simulink model "bh_TH1_CONTROL_Dual_loop_POS_SETTLE_0p05_THETA_TRACK"  (R2016b)
settings: Solver=ode23t  StartTime=0.0  StopTime=60  RelTol=1e-5  EnableMultiTasking=on
values from neighbouring files (symbols this model uses):
  g = 9.80665    [bh_params_single_link_control_explore.m]
  L1x = 1.5    [bh_params_single_link_control_explore.m]
  L1y = 0.050    (= 0.05)    [bh_params_single_link_control_explore.m]
  L1z = 0.005    [bh_params_single_link_control_explore.m]
  mass1 = density * L1x*L1y*L1z    (= 0.375)    [bh_params_single_link_control_explore.m]
undefined symbols (not defined in the file or in its folder): X, Y, Z
libraries: sm_lib x6, nesl_utility x6, simulink_extras x3, simulink x2, discretizing x1
settings Model: Creator=bhorton  LastModifiedBy=bhorton
settings SolverCC: ZeroCrossAlgorithm=Adaptive
settings OptimizationCC: LifeSpan=inf
settings DebuggingCC: SFUnexpectedBacktrackingDiag=warning  SFNoUnconditionalDefaultTransitionDiag=warning  SFExecutionAtInitializationDiag=none
settings GRTTargetCC: TargetLangStandard=C89/C90 (ANSI)
settings ConfigComp: CovMetricSettings=dw  CovHtmlReporting=on  CovSaveCumulativeToWorkspaceVar=on  CovSaveSingleToWorkspaceVar=on  CovExternalEMLEnable=off
settings SimscapeCC: SimscapeLogType=all  SimscapeLogDataHistory=10000

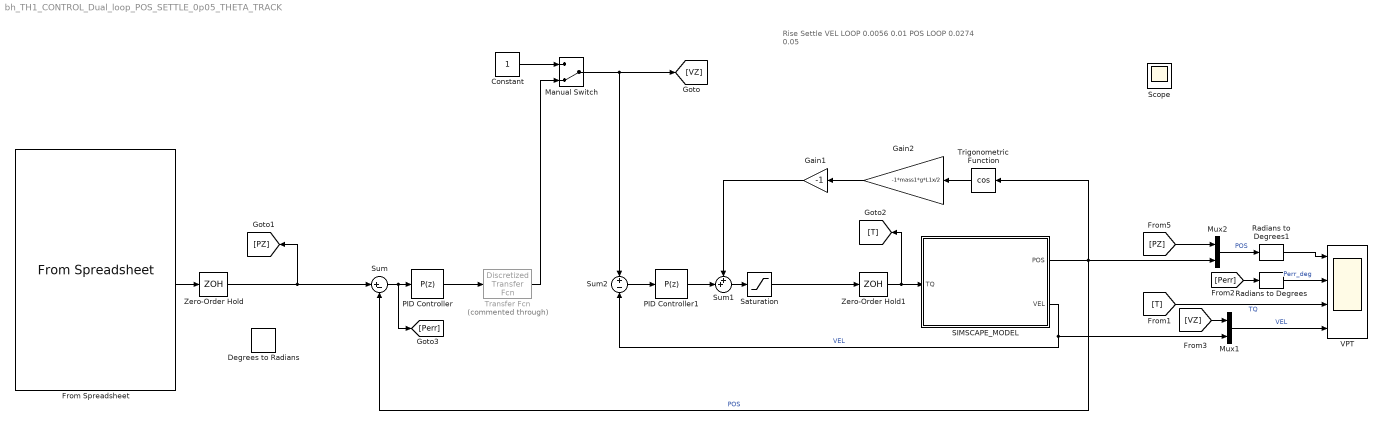
== system bh_TH1_CONTROL_Dual_loop_POS_SETTLE_0p05_THETA_TRACK ==
  note: Rise Settle
      | VEL LOOP 0.0056 0.01
      | POS LOOP 0.0274 0.05
  Constant : Constant
  Degrees to Radians : simulink_extras/Transformations/Degrees to Radians
  From Spreadsheet : FromSpreadsheet  FileName=bh_theta_data.xlsx  SheetName=THETA_SHEET  SampleTime=0.01  ExtrapolationBeforeFirstDataPoint=Hold first value  ExtrapolationAfterLastDataPoint=Hold last value
  Gain1 : Gain  Gain=-1
  Gain2 : Gain  Gain=-1*mass1*g*L1x/2
  Manual Switch : ManualSwitch  CurrentSetting=0
  Mux1 : Mux  Inputs=2
  Mux2 : Mux  Inputs=2
  PID Controller : simulink/Continuous/PID Controller  Controller=P  TimeDomain=Discrete-time  SampleTime=0.001  IntegratorMethod=Forward Euler  FilterMethod=Forward Euler  Form=Parallel  UseFilter=on  ControllerParametersSource=internal  P=63.9  I=3.94651136246193  D=0  N=100  InitialConditionSource=internal  InitialConditionForIntegrator=0  InitialConditionForFilter=0  ExternalReset=none  LimitOutput=off  UpperSaturationLimit=inf  LowerSaturationLimit=-inf  LinearizeAsGain=on  AntiWindupMode=none  Kb=1  TrackingMode=off  Kt=1  PParamMin=[]  PParamMax=[]  IParamMin=[]  IParamMax=[]  DParamMin=[]  DParamMax=[]  NParamMin=[]  NParamMax=[]  KbParamMin=[]  KbParamMax=[]  KtParamMin=[]  KtParamMax=[]  POutMin=[]  POutMax=[]  IOutMin=[]  IOutMax=[]  DOutMin=[]  DOutMax=[]  NOutMin=[]  NOutMax=[]  KbOutMin=[]  KbOutMax=[]  KtOutMin=[]  KtOutMax=[]  IntegratorOutMin=[]  IntegratorOutMax=[]  FilterOutMin=[]  FilterOutMax=[]  SumOutMin=[]  SumOutMax=[]  SumI1OutMin=[]  SumI1OutMax=[]  SumI2OutMin=[]  SumI2OutMax=[]  SumI3OutMin=[]  SumI3OutMax=[]  SumDOutMin=[]  SumDOutMax=[]  SaturationOutMin=[]  SaturationOutMax=[]  IntegratorContinuousStateAttributes=''  IntegratorStateMustResolveToSignalObject=off  IntegratorRTWStateStorageClass=Auto  FilterContinuousStateAttributes=''  FilterStateMustResolveToSignalObject=off  FilterRTWStateStorageClass=Auto  DifferentiatorICPrevScaledInput=0  DifferentiatorOutMin=[]  DifferentiatorOutMax=[]
  PID Controller1 : simulink/Continuous/PID Controller  Controller=P  TimeDomain=Discrete-time  SampleTime=0.001  IntegratorMethod=Forward Euler  FilterMethod=Forward Euler  Form=Parallel  UseFilter=on  ControllerParametersSource=internal  P=15  I=10  D=0  N=100  InitialConditionSource=internal  InitialConditionForIntegrator=0  InitialConditionForFilter=0  ExternalReset=none  LimitOutput=off  UpperSaturationLimit=inf  LowerSaturationLimit=-inf  LinearizeAsGain=on  AntiWindupMode=none  Kb=1  TrackingMode=off  Kt=1  PParamMin=[]  PParamMax=[]  IParamMin=[]  IParamMax=[]  DParamMin=[]  DParamMax=[]  NParamMin=[]  NParamMax=[]  KbParamMin=[]  KbParamMax=[]  KtParamMin=[]  KtParamMax=[]  POutMin=[]  POutMax=[]  IOutMin=[]  IOutMax=[]  DOutMin=[]  DOutMax=[]  NOutMin=[]  NOutMax=[]  KbOutMin=[]  KbOutMax=[]  KtOutMin=[]  KtOutMax=[]  IntegratorOutMin=[]  IntegratorOutMax=[]  FilterOutMin=[]  FilterOutMax=[]  SumOutMin=[]  SumOutMax=[]  SumI1OutMin=[]  SumI1OutMax=[]  SumI2OutMin=[]  SumI2OutMax=[]  SumI3OutMin=[]  SumI3OutMax=[]  SumDOutMin=[]  SumDOutMax=[]  SaturationOutMin=[]  SaturationOutMax=[]  IntegratorContinuousStateAttributes=''  IntegratorStateMustResolveToSignalObject=off  IntegratorRTWStateStorageClass=Auto  FilterContinuousStateAttributes=''  FilterStateMustResolveToSignalObject=off  FilterRTWStateStorageClass=Auto  DifferentiatorICPrevScaledInput=0  DifferentiatorOutMin=[]  DifferentiatorOutMax=[]
  Radians to Degrees : simulink_extras/Transformations/Radians to Degrees
  Radians to Degrees1 : simulink_extras/Transformations/Radians to Degrees
  SIMSCAPE_MODEL : Subsystem
  Saturation : Saturate  UpperLimit=5  LowerLimit=-5
  Sum : Sum  Inputs=|+-
  Sum1 : Sum  Inputs=++|
  Sum2 : Sum  Inputs=+|-
  Transfer Fcn : discretizing/Discretized Transfer Fcn  Commented=through  Numerator=[45]  Denominator=[1 45]  AbsTol=auto  SampleTime=0.001  method=tustin  Wc=1
  Trigonometric Function : Trigonometry  Operator=cos
  VPT : Scope  NumInputPorts=4
  Zero-Order Hold : ZeroOrderHold  SampleTime=0.001
  Zero-Order Hold1 : ZeroOrderHold  SampleTime=0.001
  Scope : Scope
  wires:
  Sum/1 -> [Perr], PID Controller/1
  From Spreadsheet/5 -> Zero-Order Hold/1
  PID Controller1/1 -> Sum1/2
  Sum1/1 -> Saturation/1
  Trigonometric Function/1 -> Gain2/1
  Gain2/1 -> Gain1/1
  Constant/1 -> Manual Switch/1
  Manual Switch/1 -> [VZ], Sum2/1
  Sum2/1 -> PID Controller1/1
  PID Controller/1 -> Transfer Fcn/1
  [VZ] -> Mux1/1
  SIMSCAPE_MODEL/1(POS) -> Sum/2, Mux2/2, Trigonometric Function/1  "POS"
  [PZ] -> Mux2/1
  SIMSCAPE_MODEL/2(VEL) -> Mux1/2, Sum2/2  "VEL"
  [T] -> VPT/3  "TQ"
  Mux2/1 -> Radians to Degrees1/1  "POS"
  Mux1/1 -> VPT/4  "VEL"
  Zero-Order Hold/1 -> [PZ], Sum/1
  Zero-Order Hold1/1 -> [T], SIMSCAPE_MODEL/1(TQ)
  Gain1/1 -> Sum1/1
  Transfer Fcn/1 -> Manual Switch/2
  Saturation/1 -> Zero-Order Hold1/1
  Radians to Degrees1/1 -> VPT/1
  [Perr] -> Radians to Degrees/1
  Radians to Degrees/1 -> VPT/2  "Perr_deg"

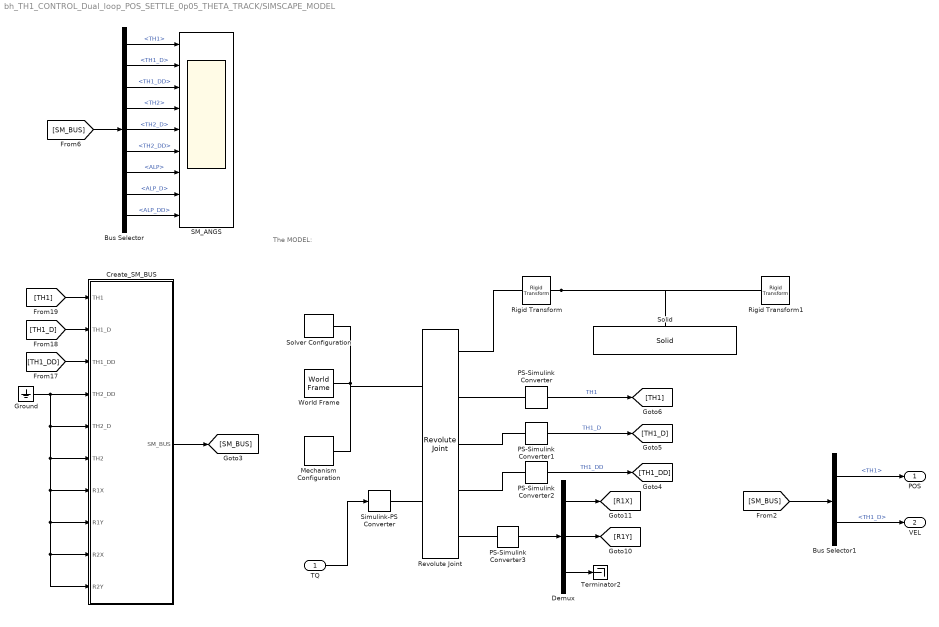
== system bh_TH1_CONTROL_Dual_loop_POS_SETTLE_0p05_THETA_TRACK/SIMSCAPE_MODEL ==
  note: The MODEL:
  TQ : Inport
  Bus Selector : BusSelector  OutputSignals=TH1,TH1_D,TH1_DD,TH2,TH2_D,TH2_DD,ALP,ALP_D,ALP_DD
  Bus Selector1 : BusSelector  OutputSignals=TH1,TH1_D
  Create_SM_BUS : Subsystem
  Demux : Demux  Outputs=3
  Ground : Ground
  Mechanism Configuration : sm_lib/Utilities/Mechanism Configuration  UniformGravity=Constant  GravityVector=[0 -9.80665 0 ]  GravityUnits=m/s^2  LinearizationDelta=0.001
  PS-Simulink Converter : nesl_utility/PS-Simulink Converter  PhysicalDomain=network_engine_domain  SubClassName=ps_output  LeftPortType=input  RightPortType=output  PseudoPeriodic=off  Frequencies=[]  Unit=rad  AffineConversion=off
  PS-Simulink Converter1 : nesl_utility/PS-Simulink Converter  PhysicalDomain=network_engine_domain  SubClassName=ps_output  LeftPortType=input  RightPortType=output  PseudoPeriodic=off  Frequencies=[]  Unit=rad/s  AffineConversion=off
  PS-Simulink Converter2 : nesl_utility/PS-Simulink Converter  PhysicalDomain=network_engine_domain  SubClassName=ps_output  LeftPortType=input  RightPortType=output  PseudoPeriodic=off  Frequencies=[]  Unit=rad/s^2  AffineConversion=off
  PS-Simulink Converter3 : nesl_utility/PS-Simulink Converter  PhysicalDomain=network_engine_domain  SubClassName=ps_output  LeftPortType=input  RightPortType=output  PseudoPeriodic=off  Frequencies=[]  Unit=N  AffineConversion=off
  Revolute Joint : sm_lib/Joints/Revolute Joint  SenseConstraintForce=on  SenseConstraintForceX=off  SenseConstraintForceY=off  SenseConstraintForceZ=off  SenseConstraintTorque=off  SenseConstraintTorqueX=off  SenseConstraintTorqueY=off  SenseConstraintTorqueZ=off  SenseTotalForce=off  SenseTotalForceX=off  SenseTotalForceY=off  SenseTotalForceZ=off  SenseTotalTorque=off  SenseTotalTorqueX=off  SenseTotalTorqueY=off  SenseTotalTorqueZ=off  CompositeWrenchDir=BaseOnFollower  CompositeWrenchFrame=BaseFrame  EquilibriumPosition=0  EquilibriumPositionUnits=deg  SpringStiffness=0  SpringStiffnessUnits=N*m/deg  DampingCoefficient=b1_damp  DampingCoefficientUnits=N*m/(rad/s)  TorqueActuationMode=InputTorque  MotionActuationMode=ComputedMotion  SensePosition=on  SenseVelocity=on  SenseAcceleration=on  SenseTorqueForce=off  PositionTargetSpecify=on  PositionTargetPriority=Low  PositionTargetValue=theta1_0  PositionTargetValueUnits=rad  VelocityTargetSpecify=on  VelocityTargetPriority=High  VelocityTargetValue=theta1_dot_0  VelocityTargetValueUnits=rad/s
  Rigid Transform : sm_lib/Frames and Transforms/Rigid Transform  TranslationMethod=StandardAxis  TranslationStandardOffset=L1x/2  TranslationLengthUnit=m  TranslationStandardAxis=+X  TranslationCartesianOffset=[0 0 0]  TranslationROffset=0  TranslationROffsetUnits=m  TranslationZOffset=0  TranslationZOffsetUnits=m  TranslationThetaOffset=0  TranslationThetaOffsetUnits=deg  RotationMethod=None  RotationAngleUnits=deg  RotationStandardAxis=+Z  RotationAngle=0.0  RotationArbitraryAxis=[0 0 1]  FollAlignAxisA=+X  BaseAlignAxisA=+Y  FollAlignAxisB=+Y  BaseAlignAxisB=+Z  RotationSequenceAxes=FollowerAxes  RotationSequence=XYX  RotationSequenceAngles=[0 0 0]  RotationSequenceAnglesUnits=deg  RotationMatrix=[1 0 0; 0 1 0; 0 0 1]
  Rigid Transform1 : sm_lib/Frames and Transforms/Rigid Transform  TranslationMethod=StandardAxis  TranslationStandardOffset=L1x/2  TranslationLengthUnit=m  TranslationStandardAxis=+X  TranslationCartesianOffset=[0 0 0]  TranslationROffset=0  TranslationROffsetUnits=m  TranslationZOffset=0  TranslationZOffsetUnits=m  TranslationThetaOffset=0  TranslationThetaOffsetUnits=deg  RotationMethod=None  RotationAngleUnits=deg  RotationStandardAxis=+Z  RotationAngle=0.0  RotationArbitraryAxis=[0 0 1]  FollAlignAxisA=+X  BaseAlignAxisA=+Y  FollAlignAxisB=+Y  BaseAlignAxisB=+Z  RotationSequenceAxes=FollowerAxes  RotationSequence=XYX  RotationSequenceAngles=[0 0 0]  RotationSequenceAnglesUnits=deg  RotationMatrix=[1 0 0; 0 1 0; 0 0 1]
  SM_ANGS : Scope  NumInputPorts=9
  Simulink-PS Converter : nesl_utility/Simulink-PS Converter  PhysicalDomain=network_engine_domain  SubClassName=ps_input  LeftPortType=input  RightPortType=output  PseudoPeriodic=off  Frequencies=[]  NoiseDistribution=none  NoiseParameters=[]  Unit=N*m  AffineConversion=off  InputFiltering=off  SimscapeFilterOrder=1  InputFilterTimeConstant=0.001  UdotUserProvided=1
  Solid : sm_lib/Body Elements/Solid  InertiaType=CalculateFromGeometry  Mass=1  MassUnits=kg  CenterOfMass=[0 0 0]  CenterOfMassUnits=m  MomentsOfInertia=[1 1 1]  MomentsOfInertiaUnits=kg*m^2  ProductsOfInertia=[0 0 0]  ProductsOfInertiaUnits=kg*m^2  DensityBased=on  Density=density  DensityUnits=kg/(m^3)  DoExposeReferenceFrame=on  SerializedFrames=<Frames/>  GraphicType=FromGeometry  MarkerShape=Sphere  MarkerSize=10  GraphicVisPropType=SimpleVisualProperties  GraphicDiffuseColor=[0.8 0.8 1.0]  GraphicSpecularColor=[0.5 0.5 0.5 1.0]  GraphicAmbientColor=[0.15 0.15 0.15 1.0]  GraphicEmissiveColor=[0.0 0.0 0.0 1.0]  GraphicShininess=75  GraphicOpacity=1.0  GeometryShape=Brick  RectangleSize=[1 1]  RectangleSizeUnits=m  BrickDimensions=[L1x, L1y, L1z ]  BrickDimensionUnits=m  CylinderRadius=1  CylinderRadiusUnits=m  CylinderLength=1  CylinderLengthUnits=m  SphereRadius=1  SphereRadiusUnits=m  EllipsoidRadii=[1 1 1]  EllipsoidRadiiUnits=m  ExtrusionCrossSection=[1 1; -1 1; -1 -1; 1 -1]  ExtrusionCrossSectionUnits=m  ExtrusionLength=1  ExtrusionLengthUnits=m  PolygonNumSides=3  PolygonOuterRadius=1  PolygonOuterRadiusUnits=m  ExtGeomFileType=STEP  ExtGeomFileUnits=m  RevolutionCrossSection=[1 1; 1 -1; 2 -1; 2 1]  RevolutionCrossSectionUnits=m  RevolutionExtent=Full  RevolutionAngle=180  RevolutionAngleUnits=deg
  Solver Configuration : nesl_utility/Solver Configuration  PhysicalDomain=network_engine_domain  SubClassName=solver  LeftPortType=input  RightPortType=generic  Accelerate=off  Tones=[]  Harmonics=[]  SimulateNoise=off  Profile=off  UseLocalSampling=off  EnableSwitchedLinearOptims=on  FrequencyDomain=off  UseCCode=off  RelTol=0.001  AbsTol=1e-06  MinStep=1e-09  ToWorkspace=off  RevertToSquareIcSolve=off  NumHomotopyIterations=100  PhasorMode=off  PhasorModeNumHarmonics=1  OverrideAbsTol=off  DoDC=off  ResidualTolerance=1e-09  UseLocalSolver=off  LocalSolverChoice=NE_BACKWARD_EULER_ADVANCER  LocalSolverSampleTime=0.001  DoFixedCost=off  MaxNonlinIter=3  MaxModeIter=2  LinearAlgebra=Sparse  DelaysMemoryBudget=1024  AutomaticFiltering=on  FilteringTimeConstant=0.001
  Terminator2 : Terminator
  World Frame : sm_lib/Frames and Transforms/World Frame
  POS : Outport
  VEL : Outport  Port=2
  wires:
  [TH1_D] -> Create_SM_BUS/2(TH1_D)
  [TH1_DD] -> Create_SM_BUS/3(TH1_DD)
  [TH1] -> Create_SM_BUS/1(TH1)
  Create_SM_BUS/1(SM_BUS) -> [SM_BUS]
  [SM_BUS] -> Bus Selector/1
  Bus Selector/2 -> SM_ANGS/2  "<TH1_D>"
  Bus Selector/3 -> SM_ANGS/3  "<TH1_DD>"
  Bus Selector/1 -> SM_ANGS/1  "<TH1>"
  Bus Selector/4 -> SM_ANGS/4  "<TH2>"
  Bus Selector/5 -> SM_ANGS/5  "<TH2_D>"
  Bus Selector/6 -> SM_ANGS/6  "<TH2_DD>"
  Bus Selector/7 -> SM_ANGS/7  "<ALP>"
  Bus Selector/8 -> SM_ANGS/8  "<ALP_D>"
  Bus Selector/9 -> SM_ANGS/9  "<ALP_DD>"
  Ground/1 -> Create_SM_BUS/5(TH2_D), Create_SM_BUS/6(TH2), Create_SM_BUS/7(R1X), Create_SM_BUS/8(R1Y), Create_SM_BUS/9(R2X), Create_SM_BUS/10(R2Y), Create_SM_BUS/4(TH2_DD)
  PS-Simulink Converter/1 -> [TH1]  "TH1"
  PS-Simulink Converter2/1 -> [TH1_DD]  "TH1_DD"
  PS-Simulink Converter1/1 -> [TH1_D]  "TH1_D"
  PS-Simulink Converter3/1 -> Demux/1
  Demux/2 -> [R1Y]
  Demux/1 -> [R1X]
  Demux/3 -> Terminator2/1
  TQ/1 -> Simulink-PS Converter/1
  [SM_BUS] -> Bus Selector1/1
  Bus Selector1/2 -> VEL/1  "<TH1_D>"
  Bus Selector1/1 -> POS/1  "<TH1>"
  connections:
  World Frame/RConn1 -- Revolute Joint/LConn1 -- Mechanism Configuration/RConn1 -- Solver Configuration/RConn1
  Rigid Transform/RConn1 -- Solid/RConn1 -- Rigid Transform1/LConn1
  Rigid Transform/LConn1 -- Revolute Joint/RConn1
  PS-Simulink Converter/LConn1 -- Revolute Joint/RConn2
  PS-Simulink Converter3/LConn1 -- Revolute Joint/RConn5
  Revolute Joint/RConn3 -- PS-Simulink Converter1/LConn1
  Revolute Joint/RConn4 -- PS-Simulink Converter2/LConn1
  Simulink-PS Converter/RConn1 -- Revolute Joint/LConn2

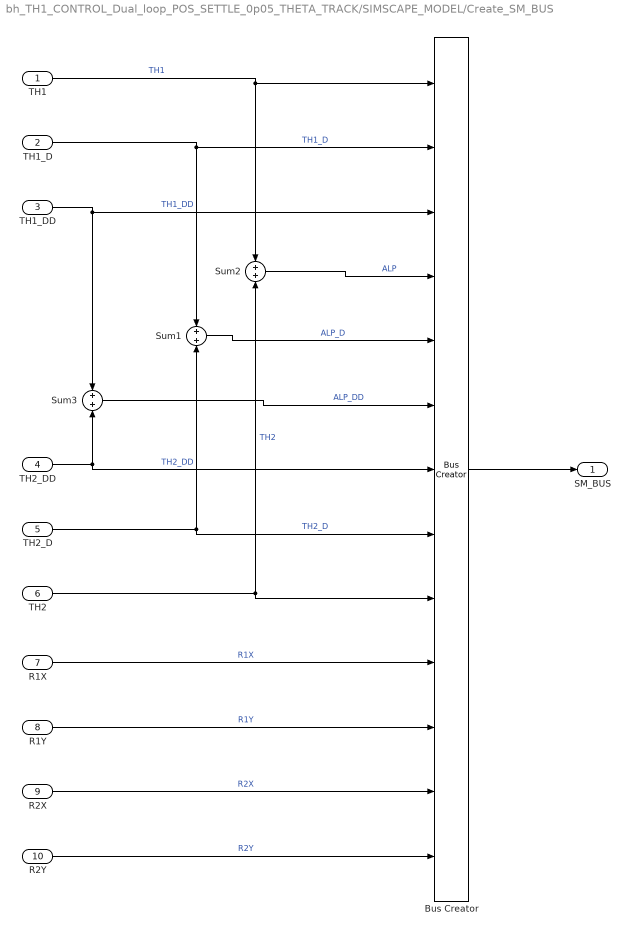
== system bh_TH1_CONTROL_Dual_loop_POS_SETTLE_0p05_THETA_TRACK/SIMSCAPE_MODEL/Create_SM_BUS ==
  TH1 : Inport
  TH1_D : Inport  Port=2
  TH1_DD : Inport  Port=3
  TH2_DD : Inport  Port=4
  TH2_D : Inport  Port=5
  TH2 : Inport  Port=6
  R1X : Inport  Port=7
  R1Y : Inport  Port=8
  R2X : Inport  Port=9
  R2Y : Inport  Port=10
  Bus Creator : BusCreator  Inputs=13
  Sum1 : Sum  Inputs=+|+
  Sum2 : Sum  Inputs=+|+
  Sum3 : Sum  Inputs=+|+
  SM_BUS : Outport
  wires:
  TH2_DD/1 -> Bus Creator/7, Sum3/2  "TH2_DD"
  TH1_DD/1 -> Sum3/1, Bus Creator/3  "TH1_DD"
  TH1_D/1 -> Bus Creator/2, Sum1/1  "TH1_D"
  TH2_D/1 -> Bus Creator/8, Sum1/2  "TH2_D"
  TH1/1 -> Bus Creator/1, Sum2/1  "TH1"
  TH2/1 -> Bus Creator/9, Sum2/2  "TH2"
  Sum2/1 -> Bus Creator/4  "ALP"
  Sum1/1 -> Bus Creator/5  "ALP_D"
  Sum3/1 -> Bus Creator/6  "ALP_DD"
  Bus Creator/1 -> SM_BUS/1
  R1Y/1 -> Bus Creator/11  "R1Y"
  R1X/1 -> Bus Creator/10  "R1X"
  R2Y/1 -> Bus Creator/13  "R2Y"
  R2X/1 -> Bus Creator/12  "R2X"
